simulink model "Q03_PED"  (Simulink 7.3)
settings: Solver=ode45  StartTime=0.0  StopTime=40  FixedStep=0.0042  RelTol=1e-10
values from neighbouring files (symbols this model uses):
  c1 = 2.94    [prelab03.m]
  k1 = 338.6    [prelab03.m]
  kd = 0.01    [prelab03.m]
  khw = 14732    [prelab03.m]
  kp = 0.08    [prelab03.m]
  kv = 0.005    [prelab03.m]
  m1 = mc1 + mw1    (= 2.778)    [prelab03.m]
libraries: simulink_extras x2
settings Model: Creator=Giovani  LastModifiedBy=Giovani

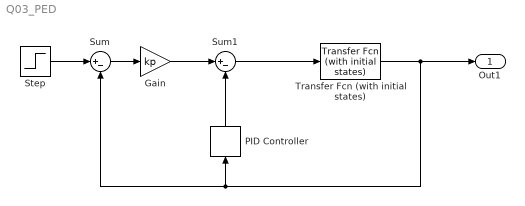
== system Q03_PED ==
  Gain : Gain  Gain=kp  ParameterDataType=fixdt(1, 16)  ParameterScaling=2^0  OutDataType=fixdt(1, 16)  OutScaling=2^0
  PID Controller : simulink_extras/Additional Linear/PID Controller  SystemSampleTime=-1  P=0  I=0  D=kd
  Step : Step  After=2500  SampleTime=0
  Sum : Sum  Inputs=|+-  OutDataType=fixdt(1, 16)  OutScaling=2^0
  Sum1 : Sum  Inputs=|+-  OutDataType=fixdt(1, 16)  OutScaling=2^0
  Transfer Fcn (with initial states) : simulink_extras/Additional Linear/Transfer Fcn (with initial states)  SystemSampleTime=-1  N=[khw]  D="[k1  (c1+khw*kv) m1]"  X0=0
  Out1 : Outport  OutDataType=fixdt(1, 16)  OutScaling=2^0
  wires:
  Transfer Fcn (with initial states)/1 -> Out1/1, Sum/2, PID Controller/1
  Sum1/1 -> Transfer Fcn (with initial states)/1
  Step/1 -> Sum/1
  Sum/1 -> Gain/1
  Gain/1 -> Sum1/1
  PID Controller/1 -> Sum1/2
